simulink library "dnb"  (Simulink 8.1)
settings: Solver=ode1  StartTime=0.0  StopTime=Inf  FixedStep=0.001  RelTol=1e-3
PostLoadFcn:
  | , if any(exist('dsrtsu_mdlpostloadfcn', 'file') == [2, 3, 6]), try dsrtsu_mdlpostloadfcn('Execute', bdroot); catch fprintf('Error in PostLoadFcn (dsrtsu_mdlpostloadfcn) for model "%s":\n %s\n', bdroot, lasterr); end, end,
undefined symbols (not defined in the file or in its folder): AACC_VehSpdError_kph, MACC_ACCFMLookUpDecel_mps2, ZERO_FLOAT
libraries: hcu_lib x1
settings Model: DSRTSU_INTERNAL_RTI_VER=450  DSRTSU_INTERNAL_RTI_TYPE=rti1401  Creator=AT015555  LastModifiedBy=AT015555

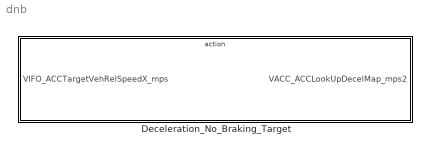
== system dnb ==
  Deceleration_No_Braking_Target : Subsystem  TreatAsAtomicUnit=on

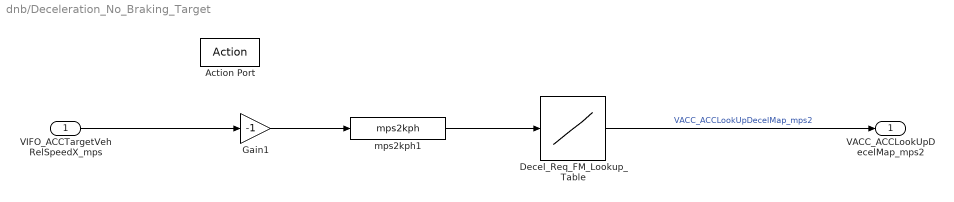
== system dnb/Deceleration_No_Braking_Target ==
  VIFO_ACCTargetVehRelSpeedX_mps : Inport
  Action Port : ActionPort
  Decel_Req_FM_Lookup_Table : Lookup_n-D  NumberOfTableDimensions=1  BreakpointsForDimension1=AACC_VehSpdError_kph  Table=MACC_ACCFMLookUpDecel_mps2  ExtrapMethod=Clip  UseLastTableValue=on  RndMeth=Simplest  InputSameDT=on
  Gain1 : Gain  Gain=-1
  mps2kph1 : hcu_lib/mps2kph
  VACC_ACCLookUpDecelMap_mps2 : Outport  OutputWhenDisabled=reset  InitialOutput=ZERO_FLOAT
  wires:
  mps2kph1/1 -> Decel_Req_FM_Lookup_Table/1
  Decel_Req_FM_Lookup_Table/1 -> VACC_ACCLookUpDecelMap_mps2/1  "VACC_ACCLookUpDecelMap_mps2"
  Gain1/1 -> mps2kph1/1
  VIFO_ACCTargetVehRelSpeedX_mps/1 -> Gain1/1
